simulink model "PP2_Q1"  (Simulink 7.9)
settings: Solver=ode45  StartTime=0.0  StopTime=15.0  RelTol=1e-3
settings Model: Creator=Basundhara  LastModifiedBy=Basundhara

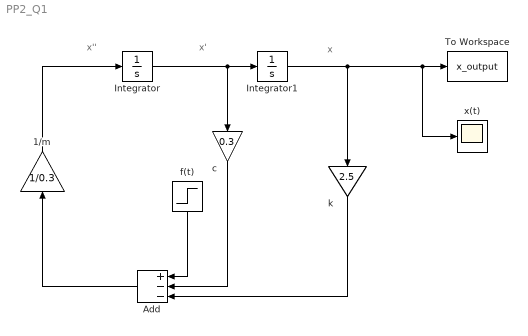
== system PP2_Q1 ==
  note: x''
  note: x'
  note: x
  1/m : Gain  Gain=1/0.3
  Add : Sum  Inputs=+--
  Integrator : Integrator
  Integrator1 : Integrator
  To Workspace : ToWorkspace  VariableName=x_output  SampleTime=-1  SaveFormat=Structure With Time
  c : Gain  Gain=0.3
  f(t) : Step  After=3  SampleTime=0
  k : Gain  Gain=2.5
  x(t) : Scope
  wires:
  f(t)/1 -> Add/1
  Integrator1/1 -> k/1, To Workspace/1, x(t)/1
  k/1 -> Add/3
  Integrator/1 -> Integrator1/1, c/1
  c/1 -> Add/2
  Add/1 -> 1/m/1
  1/m/1 -> Integrator/1
